simulink model "fir_normal"  (R2019b)
settings: Solver=VariableStepAuto  StartTime=0.0  StopTime=20000  RelTol=1e-3
undefined symbols (not defined in the file or in its folder): b
libraries: xbsIndex_r4 x52
settings Model: Creator=s4533087  LastModifiedBy=s4533087

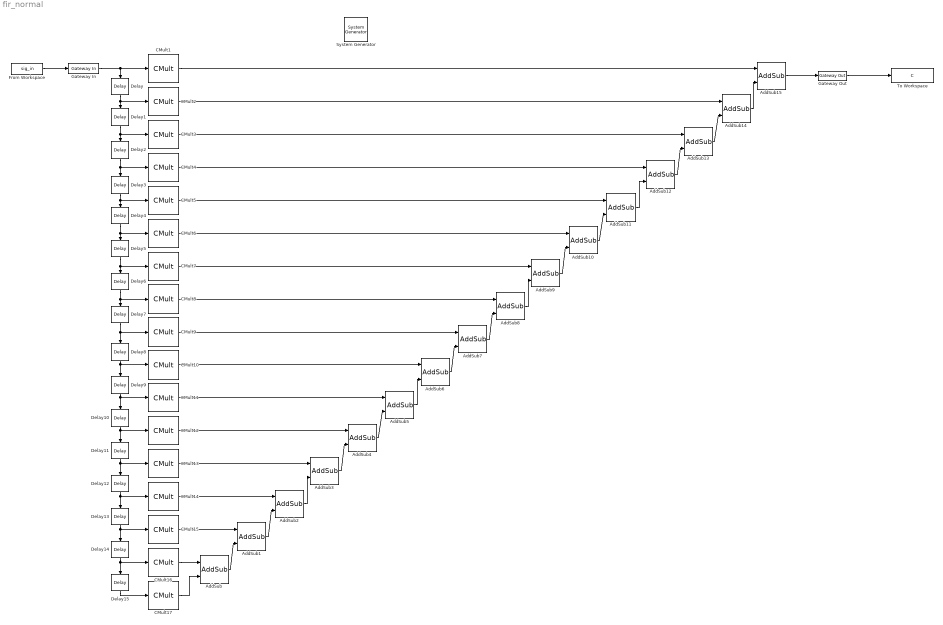
== system fir_normal ==
  " System Generator" : xbsIndex_r4/ System Generator  Tag=genX  xilinxfamily=kintex7  part=xc7k325t  speed=-3  package=fbg676  synthesis_tool=Vivado  clock_wrapper=Clock Enables  directory=./netlist  proj_type=Vivado  Synth_file=Vivado Synthesis Defaults  Impl_file=Vivado Implementation Defaults  testbench=off  simulink_period=1  sysclk_period=10  dcm_input_clock_period=10  incr_netlist=off  trim_vbits=Everywhere in SubSystem  dbl_ovrd=According to Block Masks  core_generation=According to Block Masks  run_coregen=off  deprecated_control=off  eval_field=0  block_type=sysgen
  AddSub{,1..15} (16 alike) : xbsIndex_r4/AddSub  mode=Addition  use_carryin=off  use_carryout=off  en=off  latency=0  precision=Full  arith_type=Unsigned  n_bits=16  bin_pt=14  quantization=Truncate  overflow=Wrap  use_behavioral_HDL=off  hw_selection=Fabric  pipelined=off  dbl_ovrd=off  block_type=addsub
  CMult1 : xbsIndex_r4/CMult  const=b(1)  gui_display_data_type=Fixed-point  const_n_bits=Wc  const_bin_pt=Dc  float_type=Single  exp_bits=8  fraction_bits=24  en=off  latency=1  precision=User Defined  arith_type="Signed  (2's comp)"  n_bits=Wc  bin_pt=Wc  quantization=Truncate  overflow=Wrap  use_behavioral_HDL=off  mem_type=Distributed RAM  pipeline=off  dbl_ovrd=off  block_type=cmult
  CMult10 : xbsIndex_r4/CMult  const=b(10)  gui_display_data_type=Fixed-point  const_n_bits=Wc  const_bin_pt=Dc  float_type=Single  exp_bits=8  fraction_bits=24  en=off  latency=1  precision=User Defined  arith_type="Signed  (2's comp)"  n_bits=Wc  bin_pt=Wc  quantization=Truncate  overflow=Wrap  use_behavioral_HDL=off  mem_type=Distributed RAM  pipeline=off  dbl_ovrd=off  block_type=cmult
  CMult11 : xbsIndex_r4/CMult  const=b(11)  gui_display_data_type=Fixed-point  const_n_bits=Wc  const_bin_pt=Dc  float_type=Single  exp_bits=8  fraction_bits=24  en=off  latency=1  precision=User Defined  arith_type="Signed  (2's comp)"  n_bits=Wc  bin_pt=Wc  quantization=Truncate  overflow=Wrap  use_behavioral_HDL=off  mem_type=Distributed RAM  pipeline=off  dbl_ovrd=off  block_type=cmult
  CMult12 : xbsIndex_r4/CMult  const=b(12)  gui_display_data_type=Fixed-point  const_n_bits=Wc  const_bin_pt=Dc  float_type=Single  exp_bits=8  fraction_bits=24  en=off  latency=1  precision=User Defined  arith_type="Signed  (2's comp)"  n_bits=Wc  bin_pt=Wc  quantization=Truncate  overflow=Wrap  use_behavioral_HDL=off  mem_type=Distributed RAM  pipeline=off  dbl_ovrd=off  block_type=cmult
  CMult13 : xbsIndex_r4/CMult  const=b(13)  gui_display_data_type=Fixed-point  const_n_bits=Wc  const_bin_pt=Dc  float_type=Single  exp_bits=8  fraction_bits=24  en=off  latency=1  precision=User Defined  arith_type="Signed  (2's comp)"  n_bits=Wc  bin_pt=Wc  quantization=Truncate  overflow=Wrap  use_behavioral_HDL=off  mem_type=Distributed RAM  pipeline=off  dbl_ovrd=off  block_type=cmult
  CMult14 : xbsIndex_r4/CMult  const=b(14)  gui_display_data_type=Fixed-point  const_n_bits=Wc  const_bin_pt=Dc  float_type=Single  exp_bits=8  fraction_bits=24  en=off  latency=1  precision=User Defined  arith_type="Signed  (2's comp)"  n_bits=Wc  bin_pt=Wc  quantization=Truncate  overflow=Wrap  use_behavioral_HDL=off  mem_type=Distributed RAM  pipeline=off  dbl_ovrd=off  block_type=cmult
  CMult15 : xbsIndex_r4/CMult  const=b(15)  gui_display_data_type=Fixed-point  const_n_bits=Wc  const_bin_pt=Dc  float_type=Single  exp_bits=8  fraction_bits=24  en=off  latency=1  precision=User Defined  arith_type="Signed  (2's comp)"  n_bits=Wc  bin_pt=Wc  quantization=Truncate  overflow=Wrap  use_behavioral_HDL=off  mem_type=Distributed RAM  pipeline=off  dbl_ovrd=off  block_type=cmult
  CMult16 : xbsIndex_r4/CMult  const=b(16)  gui_display_data_type=Fixed-point  const_n_bits=Wc  const_bin_pt=Dc  float_type=Single  exp_bits=8  fraction_bits=24  en=off  latency=1  precision=User Defined  arith_type="Signed  (2's comp)"  n_bits=Wc  bin_pt=Wc  quantization=Truncate  overflow=Wrap  use_behavioral_HDL=off  mem_type=Distributed RAM  pipeline=off  dbl_ovrd=off  block_type=cmult
  CMult17 : xbsIndex_r4/CMult  const=b(17)  gui_display_data_type=Fixed-point  const_n_bits=Wc  const_bin_pt=Dc  float_type=Single  exp_bits=8  fraction_bits=24  en=off  latency=1  precision=User Defined  arith_type="Signed  (2's comp)"  n_bits=Wc  bin_pt=Wc  quantization=Truncate  overflow=Wrap  use_behavioral_HDL=off  mem_type=Distributed RAM  pipeline=off  dbl_ovrd=off  block_type=cmult
  CMult2 : xbsIndex_r4/CMult  const=b(2)  gui_display_data_type=Fixed-point  const_n_bits=Wc  const_bin_pt=Dc  float_type=Single  exp_bits=8  fraction_bits=24  en=off  latency=1  precision=User Defined  arith_type="Signed  (2's comp)"  n_bits=Wc  bin_pt=Wc  quantization=Truncate  overflow=Wrap  use_behavioral_HDL=off  mem_type=Distributed RAM  pipeline=off  dbl_ovrd=off  block_type=cmult
  CMult3 : xbsIndex_r4/CMult  const=b(3)  gui_display_data_type=Fixed-point  const_n_bits=Wc  const_bin_pt=Dc  float_type=Single  exp_bits=8  fraction_bits=24  en=off  latency=1  precision=User Defined  arith_type="Signed  (2's comp)"  n_bits=Wc  bin_pt=Wc  quantization=Truncate  overflow=Wrap  use_behavioral_HDL=off  mem_type=Distributed RAM  pipeline=off  dbl_ovrd=off  block_type=cmult
  CMult4 : xbsIndex_r4/CMult  const=b(4)  gui_display_data_type=Fixed-point  const_n_bits=Wc  const_bin_pt=Dc  float_type=Single  exp_bits=8  fraction_bits=24  en=off  latency=1  precision=User Defined  arith_type="Signed  (2's comp)"  n_bits=Wc  bin_pt=Wc  quantization=Truncate  overflow=Wrap  use_behavioral_HDL=off  mem_type=Distributed RAM  pipeline=off  dbl_ovrd=off  block_type=cmult
  CMult5 : xbsIndex_r4/CMult  const=b(5)  gui_display_data_type=Fixed-point  const_n_bits=Wc  const_bin_pt=Dc  float_type=Single  exp_bits=8  fraction_bits=24  en=off  latency=1  precision=User Defined  arith_type="Signed  (2's comp)"  n_bits=Wc  bin_pt=Wc  quantization=Truncate  overflow=Wrap  use_behavioral_HDL=off  mem_type=Distributed RAM  pipeline=off  dbl_ovrd=off  block_type=cmult
  CMult6 : xbsIndex_r4/CMult  const=b(6)  gui_display_data_type=Fixed-point  const_n_bits=Wc  const_bin_pt=Dc  float_type=Single  exp_bits=8  fraction_bits=24  en=off  latency=1  precision=User Defined  arith_type="Signed  (2's comp)"  n_bits=Wc  bin_pt=Wc  quantization=Truncate  overflow=Wrap  use_behavioral_HDL=off  mem_type=Distributed RAM  pipeline=off  dbl_ovrd=off  block_type=cmult
  CMult7 : xbsIndex_r4/CMult  const=b(7)  gui_display_data_type=Fixed-point  const_n_bits=Wc  const_bin_pt=Dc  float_type=Single  exp_bits=8  fraction_bits=24  en=off  latency=1  precision=User Defined  arith_type="Signed  (2's comp)"  n_bits=Wc  bin_pt=Wc  quantization=Truncate  overflow=Wrap  use_behavioral_HDL=off  mem_type=Distributed RAM  pipeline=off  dbl_ovrd=off  block_type=cmult
  CMult8 : xbsIndex_r4/CMult  const=b(8)  gui_display_data_type=Fixed-point  const_n_bits=Wc  const_bin_pt=Dc  float_type=Single  exp_bits=8  fraction_bits=24  en=off  latency=1  precision=User Defined  arith_type="Signed  (2's comp)"  n_bits=Wc  bin_pt=Wc  quantization=Truncate  overflow=Wrap  use_behavioral_HDL=off  mem_type=Distributed RAM  pipeline=off  dbl_ovrd=off  block_type=cmult
  CMult9 : xbsIndex_r4/CMult  const=b(9)  gui_display_data_type=Fixed-point  const_n_bits=Wc  const_bin_pt=Dc  float_type=Single  exp_bits=8  fraction_bits=24  en=off  latency=1  precision=User Defined  arith_type="Signed  (2's comp)"  n_bits=Wc  bin_pt=Wc  quantization=Truncate  overflow=Wrap  use_behavioral_HDL=off  mem_type=Distributed RAM  pipeline=off  dbl_ovrd=off  block_type=cmult
  Delay{,1..15} (16 alike) : xbsIndex_r4/Delay  rst=off  infoeditControl=Selection of Reset will increase slice count due to use of real FFs and instead of SRLs  en=off  latency=1  reg_retiming=off  dbl_ovrd=off  block_type=delay
  From Workspace : FromWorkspace  VariableName=sig_in  SampleTime=0
  Gateway In : xbsIndex_r4/Gateway In  gui_display_data_type=Fixed-point  arith_type="Signed  (2's comp)"  n_bits=W  bin_pt=D  preci_type=Single  exp_width=8  frac_width=24  rows=1  columns=1  quantization="Round  (unbiased: +/- Inf)"  overflow=Saturate  period=1  UseAsADC=off  ADCChannel='1'  interface=None  automatic_assignment=on  address_offset=hex2dec('00')  intf_name=''  intf_description=''  default_value=0  timing_constraint=None  locs_specified=off  LOCs={}  io_standard={}  inherit_from_input=off  hdl_port=on  dbl_ovrd=off  block_type=gatewayin
  Gateway Out : xbsIndex_r4/Gateway Out  inherit_from_input=off  hdl_port=on  rows=1  columns=1  UseAsDAC=off  DACChannel='1'  interface=None  automatic_assignment=on  address_offset=hex2dec('00')  intf_name=''  intf_description=''  timing_constraint=None  locs_specified=off  LOCs={}  io_standard={}  block_type=gatewayout
  To Workspace : ToWorkspace  VariableName=C  SaveFormat=Timeseries  SampleTime=-1
  wires:
  From Workspace/1 -> Gateway In/1
  Delay/1 -> CMult2/1, Delay1/1
  Delay1/1 -> CMult3/1, Delay2/1
  Delay2/1 -> CMult4/1, Delay3/1
  Delay3/1 -> CMult5/1, Delay4/1
  Delay4/1 -> CMult6/1, Delay5/1
  Delay5/1 -> CMult7/1, Delay6/1
  Delay6/1 -> CMult8/1, Delay7/1
  Delay9/1 -> CMult11/1, Delay10/1
  Delay14/1 -> CMult16/1, Delay15/1
  Delay11/1 -> CMult13/1, Delay12/1
  Delay10/1 -> CMult12/1, Delay11/1
  Delay8/1 -> CMult10/1, Delay9/1
  Delay12/1 -> CMult14/1, Delay13/1
  Delay13/1 -> CMult15/1, Delay14/1
  Delay7/1 -> CMult9/1, Delay8/1
  Gateway In/1 -> CMult1/1, Delay/1
  Delay15/1 -> CMult17/1
  CMult17/1 -> AddSub/2
  CMult16/1 -> AddSub/1
  AddSub/1 -> AddSub1/2
  CMult15/1 -> AddSub1/1
  CMult14/1 -> AddSub2/1
  CMult13/1 -> AddSub3/1
  CMult12/1 -> AddSub4/1
  CMult11/1 -> AddSub5/1
  AddSub1/1 -> AddSub2/2
  AddSub2/1 -> AddSub3/2
  AddSub3/1 -> AddSub4/2
  AddSub4/1 -> AddSub5/2
  AddSub10/1 -> AddSub11/2
  AddSub6/1 -> AddSub7/2
  AddSub8/1 -> AddSub9/2
  AddSub9/1 -> AddSub10/2
  AddSub7/1 -> AddSub8/2
  AddSub12/1 -> AddSub13/2
  AddSub14/1 -> AddSub15/2
  AddSub13/1 -> AddSub14/2
  CMult10/1 -> AddSub6/1
  CMult9/1 -> AddSub7/1
  CMult8/1 -> AddSub8/1
  CMult7/1 -> AddSub9/1
  CMult6/1 -> AddSub10/1
  CMult5/1 -> AddSub11/1
  CMult4/1 -> AddSub12/1
  CMult3/1 -> AddSub13/1
  CMult2/1 -> AddSub14/1
  CMult1/1 -> AddSub15/1
  AddSub5/1 -> AddSub6/2
  AddSub11/1 -> AddSub12/2
  AddSub15/1 -> Gateway Out/1
  Gateway Out/1 -> To Workspace/1
